simulink model "counter_down"  (R2021a)
settings: Solver=FixedStepDiscrete  StartTime=0.0  StopTime=100  RelTol=1e-3  EnableMultiTasking=on
settings Model: Creator=iT-User  LastModifiedBy=iT-User
settings DataIOCC: ReturnWorkspaceOutputs=off
settings OptimizationCC: DefaultParameterBehavior=Inlined  InlineInvariantSignals=on  EnableMemcpy=off  LifeSpan=1  EfficientTunableParamExpr=on
settings DebuggingCC: UnderspecifiedInitializationDetection=Classic  MergeDetectMultiDrivingBlocksExec=none  SFMachineParentedDataDiag=warning  ArithmeticOperatorsInVariantConditions=warning
settings ModelReferenceCC: PropagateSignalLabelsOutOfModel=off
settings SFSimCC: MATLABDynamicMemAlloc=off  CustomCodeUndefinedFunction=UseInterfaceOnly
settings RTWCC: SystemTargetFile=ert.tlc  GenCodeOnly=on  TemplateMakefile=ert_default_tmf  GenerateReport=on  IncludeHyperlinkInReport=on  LaunchReport=on  GenerateTraceInfo=on  GenerateTraceReport=on  GenerateTraceReportSl=on  GenerateTraceReportSf=on  GenerateTraceReportEml=on
settings CodeAppCC: ForceParamTrailComments=on  IgnoreCustomStorageClasses=off  OperatorAnnotations=on  SimulinkDataObjDesc=on  SFDataObjDesc=on  MATLABFcnDesc=on  InsertBlockDesc=on  StateflowObjectComments=on  MATLABSourceComments=on
settings ERTTargetCC: MultiwordLength=2048  GenerateSampleERTMain=on  InlinedParameterPlacement=NonHierarchical  ERTCustomFileTemplate=example_file_process.tlc

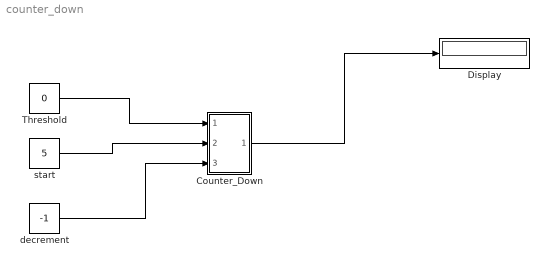
== system counter_down ==
  Counter_Down : Subsystem
  Display : Display
  Threshold : Constant  Value=0
  decrement : Constant  Value=-1
  start : Constant  Value=5
  wires:
  Threshold/1 -> Counter_Down/1(In1)
  start/1 -> Counter_Down/2(In2)
  decrement/1 -> Counter_Down/3(In3)
  Counter_Down/1(Out1) -> Display/1

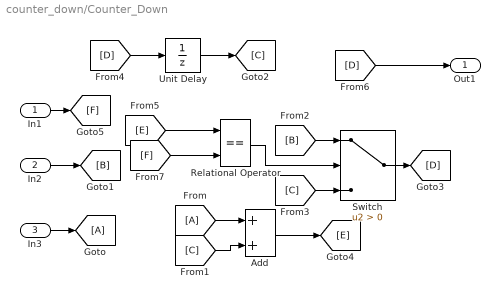
== system counter_down/Counter_Down ==
  In1 : Inport
  In2 : Inport  Port=2
  In3 : Inport  Port=3
  Add : Sum
  Relational Operator : RelationalOperator  Operator===  OutDataTypeStr=boolean  RndMeth=Simplest
  Switch : Switch  Criteria=u2 > Threshold
  Unit Delay : UnitDelay  HasFrameUpgradeWarning=on
  Out1 : Outport
  wires:
  [E] -> Relational Operator/1
  Add/1 -> [E]
  [C] -> Switch/3
  In2/1 -> [B]
  [A] -> Add/1
  [F] -> Relational Operator/2
  Unit Delay/1 -> [C]
  [D] -> Unit Delay/1
  Switch/1 -> [D]
  Relational Operator/1 -> Switch/2
  [B] -> Switch/1
  [C] -> Add/2
  In1/1 -> [F]
  In3/1 -> [A]
  [D] -> Out1/1
